simulink model "ALL_JP360_DBW_V6_5_1103"  (R2022a)
settings: Solver=FixedStepAuto  StartTime=0.0  StopTime=inf  FixedStep=0.01  RelTol=1e-3  EnableMultiTasking=on
model workspace (MAT data in the model file):
  g = 9.8
undefined symbols (not defined in the file or in its folder): canChannel, delta_v_p, IPM_Line_C0, IPM_Line_C1, IPM_Line_C2, IPM_Line_C3, M, M_p, MRR_ObjDistX, MRR_ObjDistY, MRR_ObjFusionCamID, MRR_ObjFusionSig, MRR_ObjID, MRR_ObjRelVelX, MRR_ObjRelVelY, MRR_ObjType, MRR_ObjUpdFlg, none, obj_vaild, untracktime, V, videoinput
libraries: canfdmsglib x230, canfdlib x76, slpidlib x24, simulink x18, dspstat3 x14, ctrlSharedLib x1, simulink_extras x1, imaqlib x1, realtime_pacer_lib x1, dspvision x1, visionsinks x1
(part 26 of 55)

== system ALL_JP360_DBW_V6_5_1103/MsgFromCAN/SRR_ADCU_MsgFromCAN/SRR_ADCU_FRR_OBJPos5_0x1A7 ==
  SRR_ADCU_FRR_OBJPos5_0x1A7FromInData : Inport  OutDataTypeStr=Bus:CAN_FD_MESSAGE_BUS
  Bus Creator : BusCreator  Inputs=42  OutDataTypeStr=Bus:SRR_ADCU_FRR_OBJPos5_0x1A7  NonVirtualBus=on
  CAN FD Unpack : canfdmsglib/CAN FD Unpack  CANdbFile=V363 SRR Private CAN-V1.3.dbc  MsgList=(none)  MsgName=FRR_OBJPos5_0x1A7  ProtocolMode=CAN FD  MsgIDType=Standard (11-bit identifier)  MsgIdentifier=423  MsgLength=48  SignalInfo={'FRR_CRCCheck_0x1A7','376','16','BE','unsigned','Standard','0','1','0','0','65535';'FRR_OBJ10_Dx','247','13','BE','unsigned','Standard','0','0.0625','-256','-256','255.938';'FRR_OBJ10_Dy','228','11','BE','unsigned','Standard','0','0.125','-128','-128','127.875';'FRR_OBJ10_ExistProb','280','6','BE','unsigned','Standard','0','2','0','0','100';'FRR_OBJ10_HeadingAngle','223','10','BE','unsigned','Standard','0','0.01','-3.14','-3.14','3.14';'FRR_OBJ10_Height','194','9','BE','unsigned','Standard','0','0.01','0','0','5.11';'FRR_OBJ10_Length','201','9','BE','unsigned','Standard','0','0.05','0','0','25.5';'FRR_OBJ10_Measured','294','2','BE','unsigned','Standard','0','1','0','0','3';'FRR_OBJ10_Motion_Status','330','3','BE','unsigned','Standard','0','1','0','0','7';'FRR_OBJ10_ObstacleProb','288','6','BE','unsigned','Standard','0','2','0','0','100';'FRR_OBJ10_RefPointDx','312','13','BE','unsigned','Standard','0','0.0625','-256','-256','255.938';'FRR_OBJ10_RefPointDy','309','11','BE','unsigned','Standard','0','0.125','-128','-128','127.875';'FRR_OBJ10_RefPointLoc','325','3','BE','unsigned','Standard','0','1','0','0','7';'FRR_OBJ10_RelAx','286','9','BE','unsigned','Standard','0','0.0625','-16','-16','15.9375';'FRR_OBJ10_RelAy','279','10','BE','unsigned','Standard','0','0.03125','-16','-16','15.9688';'FRR_OBJ10_RelVx','257','12','BE','unsigned','Standard','0','0.0625','-128','-128','127.938';'FRR_OBJ10_RelVy','253','10','BE','unsigned','Standard','0','0.125','-64','-64','63.875';'FRR_OBJ10_Track_Age','333','8','BE','unsigned','Standard','0','1','0','0','255';'FRR_OBJ10_Track_ID','169','7','BE','unsigned','Standard','0','1','0','0','127';'FRR_OBJ10_Type','182','3','BE','unsigned','Standard','0','1','0','0','7';'FRR_OBJ10_Width','187','11','BE','unsigned','Standard','0','0.01','0','0','12';'FRR_OBJ9_Dx','79','13','BE','unsigned','Standard','0','0.0625','-256','-256','255.938';'FRR_OBJ9_Dy','60','11','BE','unsigned','Standard','0','0.125','-128','-128','127.875';'FRR_OBJ9_ExistProb','112','6','BE','unsigned','Standard','0','2','0','0','100';'FRR_OBJ9_HeadingAngle','55','10','BE','unsigned','Standard','0','0.01','-3.14','-3.14','3.14';'FRR_OBJ9_Height','26','9','BE','unsigned','Standard','0','0.01','0','0','5.11';'FRR_OBJ9_Length','33','9','BE','unsigned','Standard','0','0.05','0','0','25.5';'FRR_OBJ9_Measured','126','2','BE','unsigned','Standard','0','1','0','0','3';'FRR_OBJ9_Motion_Status','162','3','BE','unsigned','Standard','0','1','0','0','7';'FRR_OBJ9_ObstacleProb','120','6','BE','unsigned','Standard','0','2','0','0','100';'FRR_OBJ9_RefPointDx','144','13','BE','unsigned','Standard','0','0.0625','-256','-256','255.938';'FRR_OBJ9_RefPointDy','141','11','BE','unsigned','Standard','0','0.125','-128','-128','127.875';'FRR_OBJ9_RefPointLoc','157','3','BE','unsigned','Standard','0','1','0','0','7';'FRR_OBJ9_RelAx','118','9','BE','unsigned','Standard','0','0.0625','-16','-16','15.9375';'FRR_OBJ9_RelAy','111','10','BE','unsigned','Standard','0','0.03125','-16','-16','15.9688';'FRR_OBJ9_RelVx','89','12','BE','unsigned','Standard','0','0.0625','-128','-128','127.938';'FRR_OBJ9_RelVy','85','10','BE','unsigned','Standard','0','0.125','-64','-64','63.875';'FRR_OBJ9_Track_Age','165','8','BE','unsigned','Standard','0','1','0','0','255';'FRR_OBJ9_Track_ID','1','7','BE','unsigned','Standard','0','1','0','0','127';'FRR_OBJ9_Type','14','3','BE','unsigned','Standard','0','1','0','0','7';'FRR_OBJ9_Width','19','11','BE','unsigned','Standard','0','0.01','0','0','12';'FRR_RollingCounter_0x1A7','360','4','BE','unsigned','Standard','0','1','0','0','15'}  IDPort=off  TimestampPort=off  ErrorPort=off  RemotePort=off  LengthPort=off  StatusPort=off  BRSPort=off  ESIPort=off  DLCPort=off  ApplyMinMax=off
      settings: SourceProductBaseCode=ME,XP,VN  DataFormat=CANdb specified signals
  Data Type Conversion1 : DataTypeConversion  OutDataTypeStr=uint16  SaturateOnIntegerOverflow=off  RndMeth=Floor
  Data Type Conversion{4,8..10,13,19..20,24,28..30,33,39..40,42} (15 alike) : DataTypeConversion  OutDataTypeStr=int8  SaturateOnIntegerOverflow=off  RndMeth=Floor
  Data Type Conversion{2..3,5..7,11..12,14..17,21..23,25..27,31..32,34..37,41} (24 alike) : DataTypeConversion  OutDataTypeStr=single  SaturateOnIntegerOverflow=off  RndMeth=Floor
  Data Type Conversion18 : DataTypeConversion  OutDataTypeStr=uint8  SaturateOnIntegerOverflow=off  RndMeth=Floor
  Data Type Conversion38 : DataTypeConversion  OutDataTypeStr=uint8  SaturateOnIntegerOverflow=off  RndMeth=Floor
  SRR_ADCU_FRR_OBJPos5_0x1A7FromOutData : Outport  OutDataTypeStr=Bus:SRR_ADCU_FRR_OBJPos5_0x1A7
  wires:
  CAN FD Unpack/1 -> Data Type Conversion1/1
  CAN FD Unpack/2 -> Data Type Conversion2/1
  CAN FD Unpack/3 -> Data Type Conversion3/1
  CAN FD Unpack/4 -> Data Type Conversion4/1
  CAN FD Unpack/5 -> Data Type Conversion5/1
  CAN FD Unpack/6 -> Data Type Conversion6/1
  CAN FD Unpack/7 -> Data Type Conversion7/1
  CAN FD Unpack/8 -> Data Type Conversion8/1
  CAN FD Unpack/9 -> Data Type Conversion9/1
  CAN FD Unpack/10 -> Data Type Conversion10/1
  CAN FD Unpack/11 -> Data Type Conversion11/1
  CAN FD Unpack/12 -> Data Type Conversion12/1
  CAN FD Unpack/13 -> Data Type Conversion13/1
  CAN FD Unpack/14 -> Data Type Conversion14/1
  CAN FD Unpack/15 -> Data Type Conversion15/1
  CAN FD Unpack/16 -> Data Type Conversion16/1
  CAN FD Unpack/17 -> Data Type Conversion17/1
  CAN FD Unpack/18 -> Data Type Conversion18/1
  CAN FD Unpack/19 -> Data Type Conversion19/1
  CAN FD Unpack/20 -> Data Type Conversion20/1
  CAN FD Unpack/21 -> Data Type Conversion21/1
  CAN FD Unpack/22 -> Data Type Conversion22/1
  CAN FD Unpack/23 -> Data Type Conversion23/1
  CAN FD Unpack/24 -> Data Type Conversion24/1
  CAN FD Unpack/25 -> Data Type Conversion25/1
  CAN FD Unpack/26 -> Data Type Conversion26/1
  CAN FD Unpack/27 -> Data Type Conversion27/1
  CAN FD Unpack/28 -> Data Type Conversion28/1
  CAN FD Unpack/29 -> Data Type Conversion29/1
  CAN FD Unpack/30 -> Data Type Conversion30/1
  CAN FD Unpack/31 -> Data Type Conversion31/1
  CAN FD Unpack/32 -> Data Type Conversion32/1
  CAN FD Unpack/33 -> Data Type Conversion33/1
  CAN FD Unpack/34 -> Data Type Conversion34/1
  CAN FD Unpack/35 -> Data Type Conversion35/1
  CAN FD Unpack/36 -> Data Type Conversion36/1
  CAN FD Unpack/37 -> Data Type Conversion37/1
  CAN FD Unpack/38 -> Data Type Conversion38/1
  CAN FD Unpack/39 -> Data Type Conversion39/1
  CAN FD Unpack/40 -> Data Type Conversion40/1
  CAN FD Unpack/41 -> Data Type Conversion41/1
  CAN FD Unpack/42 -> Data Type Conversion42/1
  Data Type Conversion1/1 -> Bus Creator/1  "FRR_CRCCheck_0x1A7"
  Data Type Conversion2/1 -> Bus Creator/2  "FRR_OBJ10_Dx"
  Data Type Conversion3/1 -> Bus Creator/3  "FRR_OBJ10_Dy"
  Data Type Conversion4/1 -> Bus Creator/4  "FRR_OBJ10_ExistProb"
  Data Type Conversion5/1 -> Bus Creator/5  "FRR_OBJ10_HeadingAngle"
  Data Type Conversion6/1 -> Bus Creator/6  "FRR_OBJ10_Height"
  Data Type Conversion7/1 -> Bus Creator/7  "FRR_OBJ10_Length"
  Data Type Conversion8/1 -> Bus Creator/8  "FRR_OBJ10_Measured"
  Data Type Conversion9/1 -> Bus Creator/9  "FRR_OBJ10_Motion_Status"
  Data Type Conversion10/1 -> Bus Creator/10  "FRR_OBJ10_ObstacleProb"
  Data Type Conversion11/1 -> Bus Creator/11  "FRR_OBJ10_RefPointDx"
  Data Type Conversion12/1 -> Bus Creator/12  "FRR_OBJ10_RefPointDy"
  Data Type Conversion13/1 -> Bus Creator/13  "FRR_OBJ10_RefPointLoc"
  Data Type Conversion14/1 -> Bus Creator/14  "FRR_OBJ10_RelAx"
  Data Type Conversion15/1 -> Bus Creator/15  "FRR_OBJ10_RelAy"
  Data Type Conversion16/1 -> Bus Creator/16  "FRR_OBJ10_RelVx"
  Data Type Conversion17/1 -> Bus Creator/17  "FRR_OBJ10_RelVy"
  Data Type Conversion18/1 -> Bus Creator/18  "FRR_OBJ10_Track_Age"
  Data Type Conversion19/1 -> Bus Creator/19  "FRR_OBJ10_Track_ID"
  Data Type Conversion20/1 -> Bus Creator/20  "FRR_OBJ10_Type"
  Data Type Conversion21/1 -> Bus Creator/21  "FRR_OBJ10_Width"
  Data Type Conversion22/1 -> Bus Creator/22  "FRR_OBJ9_Dx"
  Data Type Conversion23/1 -> Bus Creator/23  "FRR_OBJ9_Dy"
  Data Type Conversion24/1 -> Bus Creator/24  "FRR_OBJ9_ExistProb"
  Data Type Conversion25/1 -> Bus Creator/25  "FRR_OBJ9_HeadingAngle"
  Data Type Conversion26/1 -> Bus Creator/26  "FRR_OBJ9_Height"
  Data Type Conversion27/1 -> Bus Creator/27  "FRR_OBJ9_Length"
  Data Type Conversion28/1 -> Bus Creator/28  "FRR_OBJ9_Measured"
  Data Type Conversion29/1 -> Bus Creator/29  "FRR_OBJ9_Motion_Status"
  Data Type Conversion30/1 -> Bus Creator/30  "FRR_OBJ9_ObstacleProb"
  Data Type Conversion31/1 -> Bus Creator/31  "FRR_OBJ9_RefPointDx"
  Data Type Conversion32/1 -> Bus Creator/32  "FRR_OBJ9_RefPointDy"
  Data Type Conversion33/1 -> Bus Creator/33  "FRR_OBJ9_RefPointLoc"
  Data Type Conversion34/1 -> Bus Creator/34  "FRR_OBJ9_RelAx"
  Data Type Conversion35/1 -> Bus Creator/35  "FRR_OBJ9_RelAy"
  Data Type Conversion36/1 -> Bus Creator/36  "FRR_OBJ9_RelVx"
  Data Type Conversion37/1 -> Bus Creator/37  "FRR_OBJ9_RelVy"
  Data Type Conversion38/1 -> Bus Creator/38  "FRR_OBJ9_Track_Age"
  Data Type Conversion39/1 -> Bus Creator/39  "FRR_OBJ9_Track_ID"
  Data Type Conversion40/1 -> Bus Creator/40  "FRR_OBJ9_Type"
  Data Type Conversion41/1 -> Bus Creator/41  "FRR_OBJ9_Width"
  Data Type Conversion42/1 -> Bus Creator/42  "FRR_RollingCounter_0x1A7"
  Bus Creator/1 -> SRR_ADCU_FRR_OBJPos5_0x1A7FromOutData/1  "SRR_ADCU_FRR_OBJPos5_0x1A7FromOutData"
  SRR_ADCU_FRR_OBJPos5_0x1A7FromInData/1 -> CAN FD Unpack/1  "SRR_ADCU_FRR_OBJPos5_0x1A7FromInData"

== system ALL_JP360_DBW_V6_5_1103/MsgFromCAN/SRR_ADCU_MsgFromCAN/SRR_ADCU_FRR_OBJPos6_0x1A8 ==
  SRR_ADCU_FRR_OBJPos6_0x1A8FromInData : Inport  OutDataTypeStr=Bus:CAN_FD_MESSAGE_BUS
  Bus Creator : BusCreator  Inputs=42  OutDataTypeStr=Bus:SRR_ADCU_FRR_OBJPos6_0x1A8  NonVirtualBus=on
  CAN FD Unpack : canfdmsglib/CAN FD Unpack  CANdbFile=V363 SRR Private CAN-V1.3.dbc  MsgList=(none)  MsgName=FRR_OBJPos6_0x1A8  ProtocolMode=CAN FD  MsgIDType=Standard (11-bit identifier)  MsgIdentifier=424  MsgLength=48  SignalInfo={'FRR_CRCCheck_0x1A8','376','16','BE','unsigned','Standard','0','1','0','0','65535';'FRR_OBJ11_Dx','79','13','BE','unsigned','Standard','0','0.0625','-256','-256','255.938';'FRR_OBJ11_Dy','60','11','BE','unsigned','Standard','0','0.125','-128','-128','127.875';'FRR_OBJ11_ExistProb','112','6','BE','unsigned','Standard','0','2','0','0','100';'FRR_OBJ11_HeadingAngle','55','10','BE','unsigned','Standard','0','0.01','-3.14','-3.14','3.14';'FRR_OBJ11_Height','26','9','BE','unsigned','Standard','0','0.01','0','0','5.11';'FRR_OBJ11_Length','33','9','BE','unsigned','Standard','0','0.05','0','0','25.5';'FRR_OBJ11_Measured','126','2','BE','unsigned','Standard','0','1','0','0','3';'FRR_OBJ11_Motion_Status','162','3','BE','unsigned','Standard','0','1','0','0','7';'FRR_OBJ11_ObstacleProb','120','6','BE','unsigned','Standard','0','2','0','0','100';'FRR_OBJ11_RefPointDx','144','13','BE','unsigned','Standard','0','0.0625','-256','-256','255.938';'FRR_OBJ11_RefPointDy','141','11','BE','unsigned','Standard','0','0.125','-128','-128','127.875';'FRR_OBJ11_RefPointLoc','157','3','BE','unsigned','Standard','0','1','0','0','7';'FRR_OBJ11_RelAx','118','9','BE','unsigned','Standard','0','0.0625','-16','-16','15.9375';'FRR_OBJ11_RelAy','111','10','BE','unsigned','Standard','0','0.03125','-16','-16','15.9688';'FRR_OBJ11_RelVx','89','12','BE','unsigned','Standard','0','0.0625','-128','-128','127.938';'FRR_OBJ11_RelVy','85','10','BE','unsigned','Standard','0','0.125','-64','-64','63.875';'FRR_OBJ11_Track_Age','165','8','BE','unsigned','Standard','0','1','0','0','255';'FRR_OBJ11_Track_ID','1','7','BE','unsigned','Standard','0','1','0','0','127';'FRR_OBJ11_Type','14','3','BE','unsigned','Standard','0','1','0','0','7';'FRR_OBJ11_Width','19','11','BE','unsigned','Standard','0','0.01','0','0','12';'FRR_OBJ12_Dx','247','13','BE','unsigned','Standard','0','0.0625','-256','-256','255.938';'FRR_OBJ12_Dy','228','11','BE','unsigned','Standard','0','0.125','-128','-128','127.875';'FRR_OBJ12_ExistProb','280','6','BE','unsigned','Standard','0','2','0','0','100';'FRR_OBJ12_HeadingAngle','223','10','BE','unsigned','Standard','0','0.01','-3.14','-3.14','3.14';'FRR_OBJ12_Height','194','9','BE','unsigned','Standard','0','0.01','0','0','5.11';'FRR_OBJ12_Length','201','9','BE','unsigned','Standard','0','0.05','0','0','25.5';'FRR_OBJ12_Measured','294','2','BE','unsigned','Standard','0','1','0','0','3';'FRR_OBJ12_Motion_Status','330','3','BE','unsigned','Standard','0','1','0','0','7';'FRR_OBJ12_ObstacleProb','288','6','BE','unsigned','Standard','0','2','0','0','100';'FRR_OBJ12_RefPointDx','312','13','BE','unsigned','Standard','0','0.0625','-256','-256','255.938';'FRR_OBJ12_RefPointDy','309','11','BE','unsigned','Standard','0','0.125','-128','-128','127.875';'FRR_OBJ12_RefPointLoc','325','3','BE','unsigned','Standard','0','1','0','0','7';'FRR_OBJ12_RelAx','286','9','BE','unsigned','Standard','0','0.0625','-16','-16','15.9375';'FRR_OBJ12_RelAy','279','10','BE','unsigned','Standard','0','0.03125','-16','-16','15.9688';'FRR_OBJ12_RelVx','257','12','BE','unsigned','Standard','0','0.0625','-128','-128','127.938';'FRR_OBJ12_RelVy','253','10','BE','unsigned','Standard','0','0.125','-64','-64','63.875';'FRR_OBJ12_Track_Age','333','8','BE','unsigned','Standard','0','1','0','0','255';'FRR_OBJ12_Track_ID','169','7','BE','unsigned','Standard','0','1','0','0','127';'FRR_OBJ12_Type','182','3','BE','unsigned','Standard','0','1','0','0','7';'FRR_OBJ12_Width','187','11','BE','unsigned','Standard','0','0.01','0','0','12';'FRR_RollingCounter_0x1A8','360','4','BE','unsigned','Standard','0','1','0','0','15'}  IDPort=off  TimestampPort=off  ErrorPort=off  RemotePort=off  LengthPort=off  StatusPort=off  BRSPort=off  ESIPort=off  DLCPort=off  ApplyMinMax=off
      settings: SourceProductBaseCode=ME,XP,VN  DataFormat=CANdb specified signals
  Data Type Conversion1 : DataTypeConversion  OutDataTypeStr=uint16  SaturateOnIntegerOverflow=off  RndMeth=Floor
  Data Type Conversion{4,8..10,13,19..20,24,28..30,33,39..40,42} (15 alike) : DataTypeConversion  OutDataTypeStr=int8  SaturateOnIntegerOverflow=off  RndMeth=Floor
  Data Type Conversion{2..3,5..7,11..12,14..17,21..23,25..27,31..32,34..37,41} (24 alike) : DataTypeConversion  OutDataTypeStr=single  SaturateOnIntegerOverflow=off  RndMeth=Floor
  Data Type Conversion18 : DataTypeConversion  OutDataTypeStr=uint8  SaturateOnIntegerOverflow=off  RndMeth=Floor
  Data Type Conversion38 : DataTypeConversion  OutDataTypeStr=uint8  SaturateOnIntegerOverflow=off  RndMeth=Floor
  SRR_ADCU_FRR_OBJPos6_0x1A8FromOutData : Outport  OutDataTypeStr=Bus:SRR_ADCU_FRR_OBJPos6_0x1A8
  wires:
  CAN FD Unpack/1 -> Data Type Conversion1/1
  CAN FD Unpack/2 -> Data Type Conversion2/1
  CAN FD Unpack/3 -> Data Type Conversion3/1
  CAN FD Unpack/4 -> Data Type Conversion4/1
  CAN FD Unpack/5 -> Data Type Conversion5/1
  CAN FD Unpack/6 -> Data Type Conversion6/1
  CAN FD Unpack/7 -> Data Type Conversion7/1
  CAN FD Unpack/8 -> Data Type Conversion8/1
  CAN FD Unpack/9 -> Data Type Conversion9/1
  CAN FD Unpack/10 -> Data Type Conversion10/1
  CAN FD Unpack/11 -> Data Type Conversion11/1
  CAN FD Unpack/12 -> Data Type Conversion12/1
  CAN FD Unpack/13 -> Data Type Conversion13/1
  CAN FD Unpack/14 -> Data Type Conversion14/1
  CAN FD Unpack/15 -> Data Type Conversion15/1
  CAN FD Unpack/16 -> Data Type Conversion16/1
  CAN FD Unpack/17 -> Data Type Conversion17/1
  CAN FD Unpack/18 -> Data Type Conversion18/1
  CAN FD Unpack/19 -> Data Type Conversion19/1
  CAN FD Unpack/20 -> Data Type Conversion20/1
  CAN FD Unpack/21 -> Data Type Conversion21/1
  CAN FD Unpack/22 -> Data Type Conversion22/1
  CAN FD Unpack/23 -> Data Type Conversion23/1
  CAN FD Unpack/24 -> Data Type Conversion24/1
  CAN FD Unpack/25 -> Data Type Conversion25/1
  CAN FD Unpack/26 -> Data Type Conversion26/1
  CAN FD Unpack/27 -> Data Type Conversion27/1
  CAN FD Unpack/28 -> Data Type Conversion28/1
  CAN FD Unpack/29 -> Data Type Conversion29/1
  CAN FD Unpack/30 -> Data Type Conversion30/1
  CAN FD Unpack/31 -> Data Type Conversion31/1
  CAN FD Unpack/32 -> Data Type Conversion32/1
  CAN FD Unpack/33 -> Data Type Conversion33/1
  CAN FD Unpack/34 -> Data Type Conversion34/1
  CAN FD Unpack/35 -> Data Type Conversion35/1
  CAN FD Unpack/36 -> Data Type Conversion36/1
  CAN FD Unpack/37 -> Data Type Conversion37/1
  CAN FD Unpack/38 -> Data Type Conversion38/1
  CAN FD Unpack/39 -> Data Type Conversion39/1
  CAN FD Unpack/40 -> Data Type Conversion40/1
  CAN FD Unpack/41 -> Data Type Conversion41/1
  CAN FD Unpack/42 -> Data Type Conversion42/1
  Data Type Conversion1/1 -> Bus Creator/1  "FRR_CRCCheck_0x1A8"
  Data Type Conversion2/1 -> Bus Creator/2  "FRR_OBJ11_Dx"
  Data Type Conversion3/1 -> Bus Creator/3  "FRR_OBJ11_Dy"
  Data Type Conversion4/1 -> Bus Creator/4  "FRR_OBJ11_ExistProb"
  Data Type Conversion5/1 -> Bus Creator/5  "FRR_OBJ11_HeadingAngle"
  Data Type Conversion6/1 -> Bus Creator/6  "FRR_OBJ11_Height"
  Data Type Conversion7/1 -> Bus Creator/7  "FRR_OBJ11_Length"
  Data Type Conversion8/1 -> Bus Creator/8  "FRR_OBJ11_Measured"
  Data Type Conversion9/1 -> Bus Creator/9  "FRR_OBJ11_Motion_Status"
  Data Type Conversion10/1 -> Bus Creator/10  "FRR_OBJ11_ObstacleProb"
  Data Type Conversion11/1 -> Bus Creator/11  "FRR_OBJ11_RefPointDx"
  Data Type Conversion12/1 -> Bus Creator/12  "FRR_OBJ11_RefPointDy"
  Data Type Conversion13/1 -> Bus Creator/13  "FRR_OBJ11_RefPointLoc"
  Data Type Conversion14/1 -> Bus Creator/14  "FRR_OBJ11_RelAx"
  Data Type Conversion15/1 -> Bus Creator/15  "FRR_OBJ11_RelAy"
  Data Type Conversion16/1 -> Bus Creator/16  "FRR_OBJ11_RelVx"
  Data Type Conversion17/1 -> Bus Creator/17  "FRR_OBJ11_RelVy"
  Data Type Conversion18/1 -> Bus Creator/18  "FRR_OBJ11_Track_Age"
  Data Type Conversion19/1 -> Bus Creator/19  "FRR_OBJ11_Track_ID"
  Data Type Conversion20/1 -> Bus Creator/20  "FRR_OBJ11_Type"
  Data Type Conversion21/1 -> Bus Creator/21  "FRR_OBJ11_Width"
  Data Type Conversion22/1 -> Bus Creator/22  "FRR_OBJ12_Dx"
  Data Type Conversion23/1 -> Bus Creator/23  "FRR_OBJ12_Dy"
  Data Type Conversion24/1 -> Bus Creator/24  "FRR_OBJ12_ExistProb"
  Data Type Conversion25/1 -> Bus Creator/25  "FRR_OBJ12_HeadingAngle"
  Data Type Conversion26/1 -> Bus Creator/26  "FRR_OBJ12_Height"
  Data Type Conversion27/1 -> Bus Creator/27  "FRR_OBJ12_Length"
  Data Type Conversion28/1 -> Bus Creator/28  "FRR_OBJ12_Measured"
  Data Type Conversion29/1 -> Bus Creator/29  "FRR_OBJ12_Motion_Status"
  Data Type Conversion30/1 -> Bus Creator/30  "FRR_OBJ12_ObstacleProb"
  Data Type Conversion31/1 -> Bus Creator/31  "FRR_OBJ12_RefPointDx"
  Data Type Conversion32/1 -> Bus Creator/32  "FRR_OBJ12_RefPointDy"
  Data Type Conversion33/1 -> Bus Creator/33  "FRR_OBJ12_RefPointLoc"
  Data Type Conversion34/1 -> Bus Creator/34  "FRR_OBJ12_RelAx"
  Data Type Conversion35/1 -> Bus Creator/35  "FRR_OBJ12_RelAy"
  Data Type Conversion36/1 -> Bus Creator/36  "FRR_OBJ12_RelVx"
  Data Type Conversion37/1 -> Bus Creator/37  "FRR_OBJ12_RelVy"
  Data Type Conversion38/1 -> Bus Creator/38  "FRR_OBJ12_Track_Age"
  Data Type Conversion39/1 -> Bus Creator/39  "FRR_OBJ12_Track_ID"
  Data Type Conversion40/1 -> Bus Creator/40  "FRR_OBJ12_Type"
  Data Type Conversion41/1 -> Bus Creator/41  "FRR_OBJ12_Width"
  Data Type Conversion42/1 -> Bus Creator/42  "FRR_RollingCounter_0x1A8"
  Bus Creator/1 -> SRR_ADCU_FRR_OBJPos6_0x1A8FromOutData/1  "SRR_ADCU_FRR_OBJPos6_0x1A8FromOutData"
  SRR_ADCU_FRR_OBJPos6_0x1A8FromInData/1 -> CAN FD Unpack/1  "SRR_ADCU_FRR_OBJPos6_0x1A8FromInData"

== system ALL_JP360_DBW_V6_5_1103/MsgFromCAN/SRR_ADCU_MsgFromCAN/SRR_ADCU_FRR_OBJPos7_0x1A9 ==
  SRR_ADCU_FRR_OBJPos7_0x1A9FromInData : Inport  OutDataTypeStr=Bus:CAN_FD_MESSAGE_BUS
  Bus Creator : BusCreator  Inputs=42  OutDataTypeStr=Bus:SRR_ADCU_FRR_OBJPos7_0x1A9  NonVirtualBus=on
  CAN FD Unpack : canfdmsglib/CAN FD Unpack  CANdbFile=V363 SRR Private CAN-V1.3.dbc  MsgList=(none)  MsgName=FRR_OBJPos7_0x1A9  ProtocolMode=CAN FD  MsgIDType=Standard (11-bit identifier)  MsgIdentifier=425  MsgLength=48  SignalInfo={'FRR_CRCCheck_0x1A9','376','16','BE','unsigned','Standard','0','1','0','0','65535';'FRR_OBJ13_Dx','79','13','BE','unsigned','Standard','0','0.0625','-256','-256','255.938';'FRR_OBJ13_Dy','60','11','BE','unsigned','Standard','0','0.125','-128','-128','127.875';'FRR_OBJ13_ExistProb','112','6','BE','unsigned','Standard','0','2','0','0','100';'FRR_OBJ13_HeadingAngle','55','10','BE','unsigned','Standard','0','0.01','-3.14','-3.14','3.14';'FRR_OBJ13_Height','26','9','BE','unsigned','Standard','0','0.01','0','0','5.11';'FRR_OBJ13_Length','33','9','BE','unsigned','Standard','0','0.05','0','0','25.5';'FRR_OBJ13_Measured','126','2','BE','unsigned','Standard','0','1','0','0','3';'FRR_OBJ13_Motion_Status','162','3','BE','unsigned','Standard','0','1','0','0','7';'FRR_OBJ13_ObstacleProb','120','6','BE','unsigned','Standard','0','2','0','0','100';'FRR_OBJ13_RefPointDx','144','13','BE','unsigned','Standard','0','0.0625','-256','-256','255.938';'FRR_OBJ13_RefPointDy','141','11','BE','unsigned','Standard','0','0.125','-128','-128','127.875';'FRR_OBJ13_RefPointLoc','157','3','BE','unsigned','Standard','0','1','0','0','7';'FRR_OBJ13_RelAx','118','9','BE','unsigned','Standard','0','0.0625','-16','-16','15.9375';'FRR_OBJ13_RelAy','111','10','BE','unsigned','Standard','0','0.03125','-16','-16','15.9688';'FRR_OBJ13_RelVx','89','12','BE','unsigned','Standard','0','0.0625','-128','-128','127.938';'FRR_OBJ13_RelVy','85','10','BE','unsigned','Standard','0','0.125','-64','-64','63.875';'FRR_OBJ13_Track_Age','165','8','BE','unsigned','Standard','0','1','0','0','255';'FRR_OBJ13_Track_ID','1','7','BE','unsigned','Standard','0','1','0','0','127';'FRR_OBJ13_Type','14','3','BE','unsigned','Standard','0','1','0','0','7';'FRR_OBJ13_Width','19','11','BE','unsigned','Standard','0','0.01','0','0','12';'FRR_OBJ14_Dx','247','13','BE','unsigned','Standard','0','0.0625','-256','-256','255.938';'FRR_OBJ14_Dy','228','11','BE','unsigned','Standard','0','0.125','-128','-128','127.875';'FRR_OBJ14_ExistProb','280','6','BE','unsigned','Standard','0','2','0','0','100';'FRR_OBJ14_HeadingAngle','223','10','BE','unsigned','Standard','0','0.01','-3.14','-3.14','3.14';'FRR_OBJ14_Height','194','9','BE','unsigned','Standard','0','0.01','0','0','5.11';'FRR_OBJ14_Length','201','9','BE','unsigned','Standard','0','0.05','0','0','25.5';'FRR_OBJ14_Measured','294','2','BE','unsigned','Standard','0','1','0','0','3';'FRR_OBJ14_Motion_Status','330','3','BE','unsigned','Standard','0','1','0','0','7';'FRR_OBJ14_ObstacleProb','288','6','BE','unsigned','Standard','0','2','0','0','100';'FRR_OBJ14_RefPointDx','312','13','BE','unsigned','Standard','0','0.0625','-256','-256','255.938';'FRR_OBJ14_RefPointDy','309','11','BE','unsigned','Standard','0','0.125','-128','-128','127.875';'FRR_OBJ14_RefPointLoc','325','3','BE','unsigned','Standard','0','1','0','0','7';'FRR_OBJ14_RelAx','286','9','BE','unsigned','Standard','0','0.0625','-16','-16','15.9375';'FRR_OBJ14_RelAy','279','10','BE','unsigned','Standard','0','0.03125','-16','-16','15.9688';'FRR_OBJ14_RelVx','257','12','BE','unsigned','Standard','0','0.0625','-128','-128','127.938';'FRR_OBJ14_RelVy','253','10','BE','unsigned','Standard','0','0.125','-64','-64','63.875';'FRR_OBJ14_Track_Age','333','8','BE','unsigned','Standard','0','1','0','0','255';'FRR_OBJ14_Track_ID','169','7','BE','unsigned','Standard','0','1','0','0','127';'FRR_OBJ14_Type','182','3','BE','unsigned','Standard','0','1','0','0','7';'FRR_OBJ14_Width','187','11','BE','unsigned','Standard','0','0.01','0','0','12';'FRR_RollingCounter_0x1A9','360','4','BE','unsigned','Standard','0','1','0','0','15'}  IDPort=off  TimestampPort=off  ErrorPort=off  RemotePort=off  LengthPort=off  StatusPort=off  BRSPort=off  ESIPort=off  DLCPort=off  ApplyMinMax=off
      settings: SourceProductBaseCode=ME,XP,VN  DataFormat=CANdb specified signals
  Data Type Conversion1 : DataTypeConversion  OutDataTypeStr=uint16  SaturateOnIntegerOverflow=off  RndMeth=Floor
  Data Type Conversion{4,8..10,13,19..20,24,28..30,33,39..40,42} (15 alike) : DataTypeConversion  OutDataTypeStr=int8  SaturateOnIntegerOverflow=off  RndMeth=Floor
  Data Type Conversion{2..3,5..7,11..12,14..17,21..23,25..27,31..32,34..37,41} (24 alike) : DataTypeConversion  OutDataTypeStr=single  SaturateOnIntegerOverflow=off  RndMeth=Floor
  Data Type Conversion18 : DataTypeConversion  OutDataTypeStr=uint8  SaturateOnIntegerOverflow=off  RndMeth=Floor
  Data Type Conversion38 : DataTypeConversion  OutDataTypeStr=uint8  SaturateOnIntegerOverflow=off  RndMeth=Floor
  SRR_ADCU_FRR_OBJPos7_0x1A9FromOutData : Outport  OutDataTypeStr=Bus:SRR_ADCU_FRR_OBJPos7_0x1A9
  wires:
  CAN FD Unpack/1 -> Data Type Conversion1/1
  CAN FD Unpack/2 -> Data Type Conversion2/1
  CAN FD Unpack/3 -> Data Type Conversion3/1
  CAN FD Unpack/4 -> Data Type Conversion4/1
  CAN FD Unpack/5 -> Data Type Conversion5/1
  CAN FD Unpack/6 -> Data Type Conversion6/1
  CAN FD Unpack/7 -> Data Type Conversion7/1
  CAN FD Unpack/8 -> Data Type Conversion8/1
  CAN FD Unpack/9 -> Data Type Conversion9/1
  CAN FD Unpack/10 -> Data Type Conversion10/1
  CAN FD Unpack/11 -> Data Type Conversion11/1
  CAN FD Unpack/12 -> Data Type Conversion12/1
  CAN FD Unpack/13 -> Data Type Conversion13/1
  CAN FD Unpack/14 -> Data Type Conversion14/1
  CAN FD Unpack/15 -> Data Type Conversion15/1
  CAN FD Unpack/16 -> Data Type Conversion16/1
  CAN FD Unpack/17 -> Data Type Conversion17/1
  CAN FD Unpack/18 -> Data Type Conversion18/1
  CAN FD Unpack/19 -> Data Type Conversion19/1
  CAN FD Unpack/20 -> Data Type Conversion20/1
  CAN FD Unpack/21 -> Data Type Conversion21/1
  CAN FD Unpack/22 -> Data Type Conversion22/1
  CAN FD Unpack/23 -> Data Type Conversion23/1
  CAN FD Unpack/24 -> Data Type Conversion24/1
  CAN FD Unpack/25 -> Data Type Conversion25/1
  CAN FD Unpack/26 -> Data Type Conversion26/1
  CAN FD Unpack/27 -> Data Type Conversion27/1
  CAN FD Unpack/28 -> Data Type Conversion28/1
  CAN FD Unpack/29 -> Data Type Conversion29/1
  CAN FD Unpack/30 -> Data Type Conversion30/1
  CAN FD Unpack/31 -> Data Type Conversion31/1
  CAN FD Unpack/32 -> Data Type Conversion32/1
  CAN FD Unpack/33 -> Data Type Conversion33/1
  CAN FD Unpack/34 -> Data Type Conversion34/1
  CAN FD Unpack/35 -> Data Type Conversion35/1
  CAN FD Unpack/36 -> Data Type Conversion36/1
  CAN FD Unpack/37 -> Data Type Conversion37/1
  CAN FD Unpack/38 -> Data Type Conversion38/1
  CAN FD Unpack/39 -> Data Type Conversion39/1
  CAN FD Unpack/40 -> Data Type Conversion40/1
  CAN FD Unpack/41 -> Data Type Conversion41/1
  CAN FD Unpack/42 -> Data Type Conversion42/1
  Data Type Conversion1/1 -> Bus Creator/1  "FRR_CRCCheck_0x1A9"
  Data Type Conversion2/1 -> Bus Creator/2  "FRR_OBJ13_Dx"
  Data Type Conversion3/1 -> Bus Creator/3  "FRR_OBJ13_Dy"
  Data Type Conversion4/1 -> Bus Creator/4  "FRR_OBJ13_ExistProb"
  Data Type Conversion5/1 -> Bus Creator/5  "FRR_OBJ13_HeadingAngle"
  Data Type Conversion6/1 -> Bus Creator/6  "FRR_OBJ13_Height"
  Data Type Conversion7/1 -> Bus Creator/7  "FRR_OBJ13_Length"
  Data Type Conversion8/1 -> Bus Creator/8  "FRR_OBJ13_Measured"
  Data Type Conversion9/1 -> Bus Creator/9  "FRR_OBJ13_Motion_Status"
  Data Type Conversion10/1 -> Bus Creator/10  "FRR_OBJ13_ObstacleProb"
  Data Type Conversion11/1 -> Bus Creator/11  "FRR_OBJ13_RefPointDx"
  Data Type Conversion12/1 -> Bus Creator/12  "FRR_OBJ13_RefPointDy"
  Data Type Conversion13/1 -> Bus Creator/13  "FRR_OBJ13_RefPointLoc"
  Data Type Conversion14/1 -> Bus Creator/14  "FRR_OBJ13_RelAx"
  Data Type Conversion15/1 -> Bus Creator/15  "FRR_OBJ13_RelAy"
  Data Type Conversion16/1 -> Bus Creator/16  "FRR_OBJ13_RelVx"
  Data Type Conversion17/1 -> Bus Creator/17  "FRR_OBJ13_RelVy"
  Data Type Conversion18/1 -> Bus Creator/18  "FRR_OBJ13_Track_Age"
  Data Type Conversion19/1 -> Bus Creator/19  "FRR_OBJ13_Track_ID"
  Data Type Conversion20/1 -> Bus Creator/20  "FRR_OBJ13_Type"
  Data Type Conversion21/1 -> Bus Creator/21  "FRR_OBJ13_Width"
  Data Type Conversion22/1 -> Bus Creator/22  "FRR_OBJ14_Dx"
  Data Type Conversion23/1 -> Bus Creator/23  "FRR_OBJ14_Dy"
  Data Type Conversion24/1 -> Bus Creator/24  "FRR_OBJ14_ExistProb"
  Data Type Conversion25/1 -> Bus Creator/25  "FRR_OBJ14_HeadingAngle"
  Data Type Conversion26/1 -> Bus Creator/26  "FRR_OBJ14_Height"
  Data Type Conversion27/1 -> Bus Creator/27  "FRR_OBJ14_Length"
  Data Type Conversion28/1 -> Bus Creator/28  "FRR_OBJ14_Measured"
  Data Type Conversion29/1 -> Bus Creator/29  "FRR_OBJ14_Motion_Status"
  Data Type Conversion30/1 -> Bus Creator/30  "FRR_OBJ14_ObstacleProb"
  Data Type Conversion31/1 -> Bus Creator/31  "FRR_OBJ14_RefPointDx"
  Data Type Conversion32/1 -> Bus Creator/32  "FRR_OBJ14_RefPointDy"
  Data Type Conversion33/1 -> Bus Creator/33  "FRR_OBJ14_RefPointLoc"
  Data Type Conversion34/1 -> Bus Creator/34  "FRR_OBJ14_RelAx"
  Data Type Conversion35/1 -> Bus Creator/35  "FRR_OBJ14_RelAy"
  Data Type Conversion36/1 -> Bus Creator/36  "FRR_OBJ14_RelVx"
  Data Type Conversion37/1 -> Bus Creator/37  "FRR_OBJ14_RelVy"
  Data Type Conversion38/1 -> Bus Creator/38  "FRR_OBJ14_Track_Age"
  Data Type Conversion39/1 -> Bus Creator/39  "FRR_OBJ14_Track_ID"
  Data Type Conversion40/1 -> Bus Creator/40  "FRR_OBJ14_Type"
  Data Type Conversion41/1 -> Bus Creator/41  "FRR_OBJ14_Width"
  Data Type Conversion42/1 -> Bus Creator/42  "FRR_RollingCounter_0x1A9"
  Bus Creator/1 -> SRR_ADCU_FRR_OBJPos7_0x1A9FromOutData/1  "SRR_ADCU_FRR_OBJPos7_0x1A9FromOutData"
  SRR_ADCU_FRR_OBJPos7_0x1A9FromInData/1 -> CAN FD Unpack/1  "SRR_ADCU_FRR_OBJPos7_0x1A9FromInData"

== system ALL_JP360_DBW_V6_5_1103/MsgFromCAN/SRR_ADCU_MsgFromCAN/SRR_ADCU_FRR_OBJPos8_0x1AA ==
  SRR_ADCU_FRR_OBJPos8_0x1AAFromInData : Inport  OutDataTypeStr=Bus:CAN_FD_MESSAGE_BUS
  Bus Creator : BusCreator  Inputs=42  OutDataTypeStr=Bus:SRR_ADCU_FRR_OBJPos8_0x1AA  NonVirtualBus=on
  CAN FD Unpack : canfdmsglib/CAN FD Unpack  CANdbFile=V363 SRR Private CAN-V1.3.dbc  MsgList=(none)  MsgName=FRR_OBJPos8_0x1AA  ProtocolMode=CAN FD  MsgIDType=Standard (11-bit identifier)  MsgIdentifier=426  MsgLength=48  SignalInfo={'FRR_CRCCheck_0x1AA','376','16','BE','unsigned','Standard','0','1','0','0','65535';'FRR_OBJ15_Dx','79','13','BE','unsigned','Standard','0','0.0625','-256','-256','255.938';'FRR_OBJ15_Dy','60','11','BE','unsigned','Standard','0','0.125','-128','-128','127.875';'FRR_OBJ15_ExistProb','112','6','BE','unsigned','Standard','0','2','0','0','100';'FRR_OBJ15_HeadingAngle','55','10','BE','unsigned','Standard','0','0.01','-3.14','-3.14','3.14';'FRR_OBJ15_Height','26','9','BE','unsigned','Standard','0','0.01','0','0','5.11';'FRR_OBJ15_Length','33','9','BE','unsigned','Standard','0','0.05','0','0','25.5';'FRR_OBJ15_Measured','126','2','BE','unsigned','Standard','0','1','0','0','3';'FRR_OBJ15_Motion_Status','162','3','BE','unsigned','Standard','0','1','0','0','7';'FRR_OBJ15_ObstacleProb','120','6','BE','unsigned','Standard','0','2','0','0','100';'FRR_OBJ15_RefPointDx','144','13','BE','unsigned','Standard','0','0.0625','-256','-256','255.938';'FRR_OBJ15_RefPointDy','141','11','BE','unsigned','Standard','0','0.125','-128','-128','127.875';'FRR_OBJ15_RefPointLoc','157','3','BE','unsigned','Standard','0','1','0','0','7';'FRR_OBJ15_RelAx','118','9','BE','unsigned','Standard','0','0.0625','-16','-16','15.9375';'FRR_OBJ15_RelAy','111','10','BE','unsigned','Standard','0','0.03125','-16','-16','15.9688';'FRR_OBJ15_RelVx','89','12','BE','unsigned','Standard','0','0.0625','-128','-128','127.938';'FRR_OBJ15_RelVy','85','10','BE','unsigned','Standard','0','0.125','-64','-64','63.875';'FRR_OBJ15_Track_Age','165','8','BE','unsigned','Standard','0','1','0','0','255';'FRR_OBJ15_Track_ID','1','7','BE','unsigned','Standard','0','1','0','0','127';'FRR_OBJ15_Type','14','3','BE','unsigned','Standard','0','1','0','0','7';'FRR_OBJ15_Width','19','11','BE','unsigned','Standard','0','0.01','0','0','12';'FRR_OBJ16_Dx','247','13','BE','unsigned','Standard','0','0.0625','-256','-256','255.938';'FRR_OBJ16_Dy','228','11','BE','unsigned','Standard','0','0.125','-128','-128','127.875';'FRR_OBJ16_ExistProb','280','6','BE','unsigned','Standard','0','2','0','0','100';'FRR_OBJ16_HeadingAngle','223','10','BE','unsigned','Standard','0','0.01','-3.14','-3.14','3.14';'FRR_OBJ16_Height','194','9','BE','unsigned','Standard','0','0.01','0','0','5.11';'FRR_OBJ16_Length','201','9','BE','unsigned','Standard','0','0.05','0','0','25.5';'FRR_OBJ16_Measured','294','2','BE','unsigned','Standard','0','1','0','0','3';'FRR_OBJ16_Motion_Status','330','3','BE','unsigned','Standard','0','1','0','0','7';'FRR_OBJ16_ObstacleProb','288','6','BE','unsigned','Standard','0','2','0','0','100';'FRR_OBJ16_RefPointDx','312','13','BE','unsigned','Standard','0','0.0625','-256','-256','255.938';'FRR_OBJ16_RefPointDy','309','11','BE','unsigned','Standard','0','0.125','-128','-128','127.875';'FRR_OBJ16_RefPointLoc','325','3','BE','unsigned','Standard','0','1','0','0','7';'FRR_OBJ16_RelAx','286','9','BE','unsigned','Standard','0','0.0625','-16','-16','15.9375';'FRR_OBJ16_RelAy','279','10','BE','unsigned','Standard','0','0.03125','-16','-16','15.9688';'FRR_OBJ16_RelVx','257','12','BE','unsigned','Standard','0','0.0625','-128','-128','127.938';'FRR_OBJ16_RelVy','253','10','BE','unsigned','Standard','0','0.125','-64','-64','63.875';'FRR_OBJ16_Track_Age','333','8','BE','unsigned','Standard','0','1','0','0','255';'FRR_OBJ16_Track_ID','169','7','BE','unsigned','Standard','0','1','0','0','127';'FRR_OBJ16_Type','182','3','BE','unsigned','Standard','0','1','0','0','7';'FRR_OBJ16_Width','187','11','BE','unsigned','Standard','0','0.01','0','0','12';'FRR_RollingCounter_0x1AA','360','4','BE','unsigned','Standard','0','1','0','0','15'}  IDPort=off  TimestampPort=off  ErrorPort=off  RemotePort=off  LengthPort=off  StatusPort=off  BRSPort=off  ESIPort=off  DLCPort=off  ApplyMinMax=off
      settings: SourceProductBaseCode=ME,XP,VN  DataFormat=CANdb specified signals
  Data Type Conversion1 : DataTypeConversion  OutDataTypeStr=uint16  SaturateOnIntegerOverflow=off  RndMeth=Floor
  Data Type Conversion{4,8..10,13,19..20,24,28..30,33,39..40,42} (15 alike) : DataTypeConversion  OutDataTypeStr=int8  SaturateOnIntegerOverflow=off  RndMeth=Floor
  Data Type Conversion{2..3,5..7,11..12,14..17,21..23,25..27,31..32,34..37,41} (24 alike) : DataTypeConversion  OutDataTypeStr=single  SaturateOnIntegerOverflow=off  RndMeth=Floor
  Data Type Conversion18 : DataTypeConversion  OutDataTypeStr=uint8  SaturateOnIntegerOverflow=off  RndMeth=Floor
  Data Type Conversion38 : DataTypeConversion  OutDataTypeStr=uint8  SaturateOnIntegerOverflow=off  RndMeth=Floor
  SRR_ADCU_FRR_OBJPos8_0x1AAFromOutData : Outport  OutDataTypeStr=Bus:SRR_ADCU_FRR_OBJPos8_0x1AA
  wires:
  CAN FD Unpack/1 -> Data Type Conversion1/1
  CAN FD Unpack/2 -> Data Type Conversion2/1
  CAN FD Unpack/3 -> Data Type Conversion3/1
  CAN FD Unpack/4 -> Data Type Conversion4/1
  CAN FD Unpack/5 -> Data Type Conversion5/1
  CAN FD Unpack/6 -> Data Type Conversion6/1
  CAN FD Unpack/7 -> Data Type Conversion7/1
  CAN FD Unpack/8 -> Data Type Conversion8/1
  CAN FD Unpack/9 -> Data Type Conversion9/1
  CAN FD Unpack/10 -> Data Type Conversion10/1
  CAN FD Unpack/11 -> Data Type Conversion11/1
  CAN FD Unpack/12 -> Data Type Conversion12/1
  CAN FD Unpack/13 -> Data Type Conversion13/1
  CAN FD Unpack/14 -> Data Type Conversion14/1
  CAN FD Unpack/15 -> Data Type Conversion15/1
  CAN FD Unpack/16 -> Data Type Conversion16/1
  CAN FD Unpack/17 -> Data Type Conversion17/1
  CAN FD Unpack/18 -> Data Type Conversion18/1
  CAN FD Unpack/19 -> Data Type Conversion19/1
  CAN FD Unpack/20 -> Data Type Conversion20/1
  CAN FD Unpack/21 -> Data Type Conversion21/1
  CAN FD Unpack/22 -> Data Type Conversion22/1
  CAN FD Unpack/23 -> Data Type Conversion23/1
  CAN FD Unpack/24 -> Data Type Conversion24/1
  CAN FD Unpack/25 -> Data Type Conversion25/1
  CAN FD Unpack/26 -> Data Type Conversion26/1
  CAN FD Unpack/27 -> Data Type Conversion27/1
  CAN FD Unpack/28 -> Data Type Conversion28/1
  CAN FD Unpack/29 -> Data Type Conversion29/1
  CAN FD Unpack/30 -> Data Type Conversion30/1
  CAN FD Unpack/31 -> Data Type Conversion31/1
  CAN FD Unpack/32 -> Data Type Conversion32/1
  CAN FD Unpack/33 -> Data Type Conversion33/1
  CAN FD Unpack/34 -> Data Type Conversion34/1
  CAN FD Unpack/35 -> Data Type Conversion35/1
  CAN FD Unpack/36 -> Data Type Conversion36/1
  CAN FD Unpack/37 -> Data Type Conversion37/1
  CAN FD Unpack/38 -> Data Type Conversion38/1
  CAN FD Unpack/39 -> Data Type Conversion39/1
  CAN FD Unpack/40 -> Data Type Conversion40/1
  CAN FD Unpack/41 -> Data Type Conversion41/1
  CAN FD Unpack/42 -> Data Type Conversion42/1
  Data Type Conversion1/1 -> Bus Creator/1  "FRR_CRCCheck_0x1AA"
  Data Type Conversion2/1 -> Bus Creator/2  "FRR_OBJ15_Dx"
  Data Type Conversion3/1 -> Bus Creator/3  "FRR_OBJ15_Dy"
  Data Type Conversion4/1 -> Bus Creator/4  "FRR_OBJ15_ExistProb"
  Data Type Conversion5/1 -> Bus Creator/5  "FRR_OBJ15_HeadingAngle"
  Data Type Conversion6/1 -> Bus Creator/6  "FRR_OBJ15_Height"
  Data Type Conversion7/1 -> Bus Creator/7  "FRR_OBJ15_Length"
  Data Type Conversion8/1 -> Bus Creator/8  "FRR_OBJ15_Measured"
  Data Type Conversion9/1 -> Bus Creator/9  "FRR_OBJ15_Motion_Status"
  Data Type Conversion10/1 -> Bus Creator/10  "FRR_OBJ15_ObstacleProb"
  Data Type Conversion11/1 -> Bus Creator/11  "FRR_OBJ15_RefPointDx"
  Data Type Conversion12/1 -> Bus Creator/12  "FRR_OBJ15_RefPointDy"
  Data Type Conversion13/1 -> Bus Creator/13  "FRR_OBJ15_RefPointLoc"
  Data Type Conversion14/1 -> Bus Creator/14  "FRR_OBJ15_RelAx"
  Data Type Conversion15/1 -> Bus Creator/15  "FRR_OBJ15_RelAy"
  Data Type Conversion16/1 -> Bus Creator/16  "FRR_OBJ15_RelVx"
  Data Type Conversion17/1 -> Bus Creator/17  "FRR_OBJ15_RelVy"
  Data Type Conversion18/1 -> Bus Creator/18  "FRR_OBJ15_Track_Age"
  Data Type Conversion19/1 -> Bus Creator/19  "FRR_OBJ15_Track_ID"
  Data Type Conversion20/1 -> Bus Creator/20  "FRR_OBJ15_Type"
  Data Type Conversion21/1 -> Bus Creator/21  "FRR_OBJ15_Width"
  Data Type Conversion22/1 -> Bus Creator/22  "FRR_OBJ16_Dx"
  Data Type Conversion23/1 -> Bus Creator/23  "FRR_OBJ16_Dy"
  Data Type Conversion24/1 -> Bus Creator/24  "FRR_OBJ16_ExistProb"
  Data Type Conversion25/1 -> Bus Creator/25  "FRR_OBJ16_HeadingAngle"
  Data Type Conversion26/1 -> Bus Creator/26  "FRR_OBJ16_Height"
  Data Type Conversion27/1 -> Bus Creator/27  "FRR_OBJ16_Length"
  Data Type Conversion28/1 -> Bus Creator/28  "FRR_OBJ16_Measured"
  Data Type Conversion29/1 -> Bus Creator/29  "FRR_OBJ16_Motion_Status"
  Data Type Conversion30/1 -> Bus Creator/30  "FRR_OBJ16_ObstacleProb"
  Data Type Conversion31/1 -> Bus Creator/31  "FRR_OBJ16_RefPointDx"
  Data Type Conversion32/1 -> Bus Creator/32  "FRR_OBJ16_RefPointDy"
  Data Type Conversion33/1 -> Bus Creator/33  "FRR_OBJ16_RefPointLoc"
  Data Type Conversion34/1 -> Bus Creator/34  "FRR_OBJ16_RelAx"
  Data Type Conversion35/1 -> Bus Creator/35  "FRR_OBJ16_RelAy"
  Data Type Conversion36/1 -> Bus Creator/36  "FRR_OBJ16_RelVx"
  Data Type Conversion37/1 -> Bus Creator/37  "FRR_OBJ16_RelVy"
  Data Type Conversion38/1 -> Bus Creator/38  "FRR_OBJ16_Track_Age"
  Data Type Conversion39/1 -> Bus Creator/39  "FRR_OBJ16_Track_ID"
  Data Type Conversion40/1 -> Bus Creator/40  "FRR_OBJ16_Type"
  Data Type Conversion41/1 -> Bus Creator/41  "FRR_OBJ16_Width"
  Data Type Conversion42/1 -> Bus Creator/42  "FRR_RollingCounter_0x1AA"
  Bus Creator/1 -> SRR_ADCU_FRR_OBJPos8_0x1AAFromOutData/1  "SRR_ADCU_FRR_OBJPos8_0x1AAFromOutData"
  SRR_ADCU_FRR_OBJPos8_0x1AAFromInData/1 -> CAN FD Unpack/1  "SRR_ADCU_FRR_OBJPos8_0x1AAFromInData"
